simulink model "IPD"  (R2020a)
settings: Solver=VariableStepAuto  StartTime=0.0  StopTime=5  RelTol=1e-3
values from neighbouring files (symbols this model uses):
  Ac = [0, 1; -tf3.denominator{1}(3), -tf3.denominator{1}(2)]    [modelo.m]    (also in rei.m)
  Bc = [0; tf3.numerator{1}(3)]    [modelo.m]    (also in rei.m)
  Cc = [1, 0]    [modelo.m]    (also in rei.m)
  Kd = 2.5494    [control_pamh_tarea1.m]    (also in modelo.m = Kss(2))
  Ki = 2.6458    [control_pamh_tarea1.m]    (also in modelo.m = -Kss(3))
  Kp = 1.8496    [control_pamh_tarea1.m]    (also in modelo.m = Kss(1))
settings Model: Creator=jdavi  LastModifiedBy=jdavi

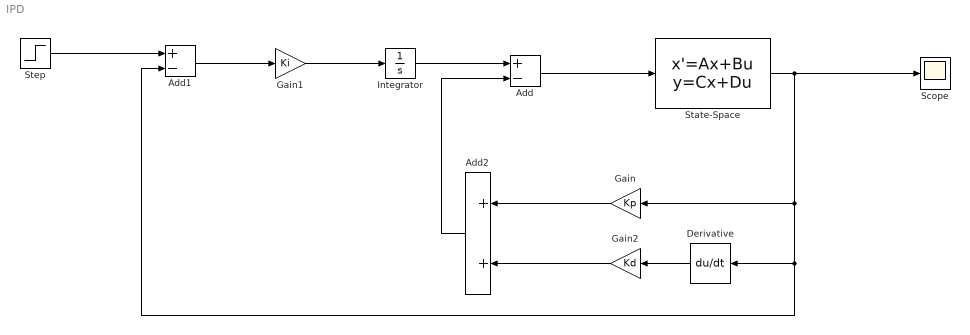
== system IPD ==
  Add : Sum  Inputs=+-
  Add1 : Sum  Inputs=+-
  Add2 : Sum
  Derivative : Derivative
  Gain : Gain  Gain=Kp
  Gain1 : Gain  Gain=Ki
  Gain2 : Gain  Gain=Kd
  Integrator : Integrator
  Scope : Scope
  State-Space : StateSpace  A=Ac  B=Bc  C=Cc  D=0  InitialCondition=0
  Step : Step  Time=0  SampleTime=0
  wires:
  Add/1 -> State-Space/1
  Gain1/1 -> Integrator/1
  Add1/1 -> Gain1/1
  Step/1 -> Add1/1
  Integrator/1 -> Add/1
  State-Space/1 -> Scope/1, Derivative/1, Add1/2, Gain/1
  Add2/1 -> Add/2
  Gain/1 -> Add2/1
  Derivative/1 -> Gain2/1
  Gain2/1 -> Add2/2
